simulink model "water_bowl"  (R2023a)
settings: Solver=VariableStepAuto  StartTime=0.0  StopTime=24  RelTol=1e-3
libraries: embmathops x2, simulink x1
settings Model: Creator=laurabryant  LastModifiedBy=umphaipunatipunumphai

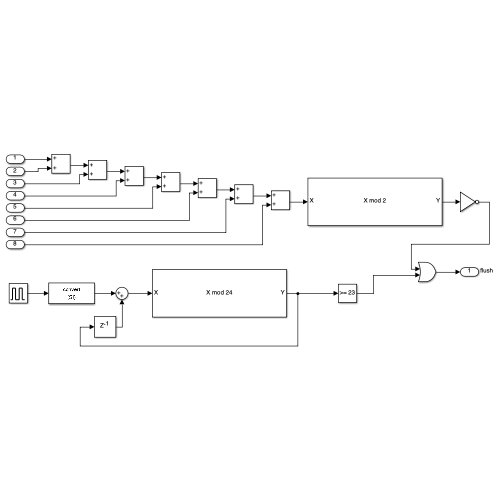
[thumbnail: Simulink's stored preview of the top-level diagram]
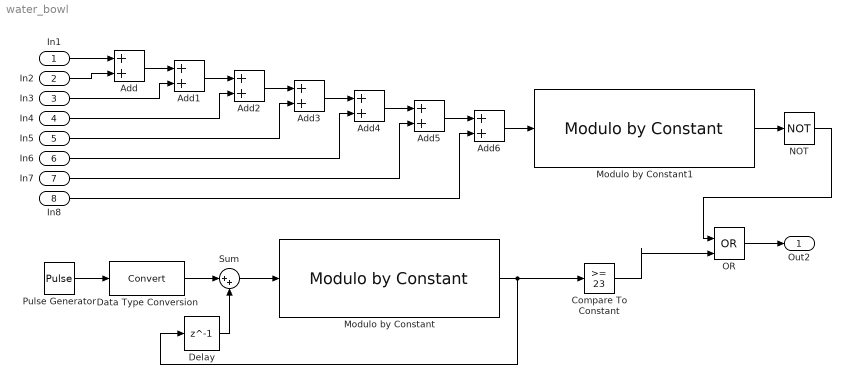
== system water_bowl ==
  In1 : Inport  OutDataTypeStr=boolean
  In2 : Inport  Port=2
  In3 : Inport  Port=3
  In4 : Inport  Port=4
  In5 : Inport  Port=5
  In6 : Inport  Port=6
  In7 : Inport  Port=7
  In8 : Inport  Port=8
  Add{,1..6} (7 alike) : Sum
  Compare To Constant : simulink/Logic and Bit Operations/Compare To Constant  relop=>=  const=23  OutDataTypeStr=boolean
  Data Type Conversion : DataTypeConversion  OutMin=0  OutMax=1  ConvertRealWorld=Stored Integer (SI)  RndMeth=Nearest  SaturateOnIntegerOverflow=off
  Delay : Delay  DelayLength=1  InitialCondition=0  SampleTime=1
  Modulo by Constant : embmathops/Modulo by Constant  Denominator=24  SimulateUsing=Code generation
      settings: LibrarySourceBlock=embeddedMathLib/Modulo by Constant
  Modulo by Constant1 : embmathops/Modulo by Constant  Denominator=2  SimulateUsing=Code generation
      settings: LibrarySourceBlock=embeddedMathLib/Modulo by Constant
  NOT : Logic  Operator=NOT  IconShape=distinctive  AllPortsSameDT=off  OutDataTypeStr=boolean
  OR : Logic  Operator=OR  IconShape=distinctive  AllPortsSameDT=off  OutDataTypeStr=boolean
  Pulse Generator : DiscretePulseGenerator  PulseType=Time based  Period=1  PulseWidth=2
  Sum : Sum  Inputs=|++
  Out2 : Outport  SignalName=flush
  wires:
  Delay/1 -> Sum/2
  Modulo by Constant/1 -> Compare To Constant/1, Delay/1
  Sum/1 -> Modulo by Constant/1
  Data Type Conversion/1 -> Sum/1
  Pulse Generator/1 -> Data Type Conversion/1
  Compare To Constant/1 -> OR/2
  OR/1 -> Out2/1
  In1/1 -> Add/1
  In2/1 -> Add/2
  Add/1 -> Add1/1
  In3/1 -> Add1/2
  Add1/1 -> Add2/1
  In4/1 -> Add2/2
  Add2/1 -> Add3/1
  In5/1 -> Add3/2
  Add3/1 -> Add4/1
  In6/1 -> Add4/2
  Add4/1 -> Add5/1
  In7/1 -> Add5/2
  Add5/1 -> Add6/1
  In8/1 -> Add6/2
  Add6/1 -> Modulo by Constant1/1
  Modulo by Constant1/1 -> NOT/1
  NOT/1 -> OR/1
